simulink model "controller_only"  (R2016a)
settings: Solver=FixedStepAuto  StartTime=0.0  StopTime=25  FixedStep=0.1  RelTol=1e-3
settings Model: ExtModeTrigDuration=5  Creator=aless  LastModifiedBy=aless
settings OptimizationCC: DefaultParameterBehavior=Inlined  OptimizeModelRefInitCode=on  LifeSpan=1
settings HardwareCC: ProdBitPerPointer=32  ProdLargestAtomicInteger=Long  ProdLargestAtomicFloat=Double  ProdWordSize=32  ProdHWDeviceType=ARM Compatible->ARM Cortex
settings RTWCC: SystemTargetFile=ert.tlc  GenCodeOnly=on  TemplateMakefile=ert_default_tmf  GenerateReport=on  IncludeHyperlinkInReport=on  LaunchReport=on  GenerateTraceInfo=on  GenerateTraceReport=on  GenerateTraceReportSl=on  GenerateTraceReportSf=on  GenerateTraceReportEml=on
settings CodeAppCC: ForceParamTrailComments=on  OperatorAnnotations=on  SimulinkDataObjDesc=on  SFDataObjDesc=on  MATLABFcnDesc=on  InsertBlockDesc=on  MATLABSourceComments=on
settings ERTTargetCC: GenerateSampleERTMain=on  MultiInstanceERTCode=on  CodeInterfacePackaging=Reusable function  InlinedParameterPlacement=NonHierarchical  RootIOFormat=Structure reference  ERTCustomFileTemplate=example_file_process.tlc  ERTFilePackagingFormat=Compact

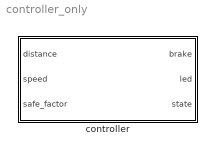
== system controller_only ==
  controller : Subsystem

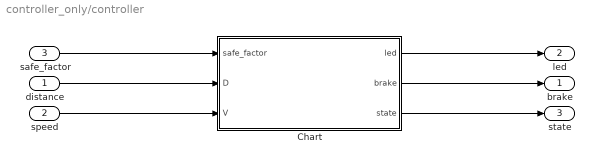
== system controller_only/controller ==
  distance : Inport
  speed : Inport  Port=2
  safe_factor : Inport  Port=3
  Chart : Stateflow chart  TreatAsAtomicUnit=on
  brake : Outport
  led : Outport  Port=2
  state : Outport  Port=3
  wires:
  distance/1 -> Chart/2(D)
  speed/1 -> Chart/3(V)
  safe_factor/1 -> Chart/1(safe_factor)
  Chart/1(led) -> led/1
  Chart/2(brake) -> brake/1
  Chart/3(state) -> state/1

== stateflow chart controller_only/controller/Chart ==
  state INIT_STATE
    en: brake = uint8(0),
    led = uint8(0),
    state = uint8(0);
  state UNSAFE_DISTANCE
    en: brake = uint8(1);
    state LED_ON
      en: led = uint8(1);
    state LED_OFF
      en: led = uint8(0);
    (default) -> LED_ON
    LED_OFF -> LED_ON : after(1/(1+V^2/100-D), msec)
    LED_ON -> LED_OFF : after(1/(1+V^2/100-D), msec)
  state SAFE_DISTANCE
    en: brake = uint8(0),
    led = uint8(0);
  (default) -> INIT_STATE
  INIT_STATE -> UNSAFE_DISTANCE [order 2] : [D <= (V^2)/100]
  INIT_STATE -> SAFE_DISTANCE [order 1] : [D > (V^2)/100]
  SAFE_DISTANCE -> UNSAFE_DISTANCE : [D <= (V^2)/100]
  UNSAFE_DISTANCE -> SAFE_DISTANCE : [D > (V^2)/100 * safe_factor]
  data: led output; safe_factor input; brake output; D input; V input; state output
